simulink model "MVP2_BVA_Control_Final_Arduino1"  (R2020a)
settings: Solver=FixedStepAuto  StartTime=0.0  StopTime=inf  FixedStep=0.01  RelTol=1e-3  EnableMultiTasking=on
PreLoadFcn:
  | Time=[
  | 0
  | 0.15
  | 0.3
  | 0.45
  | 0.6
  | 0.75
  | 0.9
  | 1.05
  | 1.2
  | 1.35
  | 1.5
  | 1.65
  | 1.8
  | 1.95
  | 2.1
  | 2.25
  | 2.4
  | 2.55
  | 2.7
  | 2.85
  | 3]
  | Output=[
  | 1
  | 1
  | 1
  | 1
  | 1
  | 1
  | 1
  | 1
  | 1
  | 1
  | 1
  | 0
  | 0
  | 0
  | 0
  | 0
  | 0
  | 0
  | 0
  | 0
  | 0];
InitFcn:
  | k=3/6;
libraries: arduinolib x13
settings Model: SILPILModeSetting=veronly  ExtModeTrigDuration=2  Creator=drlee  LastModifiedBy=drlee
settings SolverCC: AutoInsertRateTranBlk=on
settings OptimizationCC: EnhancedBackFolding=on  PassReuseOutputArgsAs=Individual arguments  ZeroExternalMemoryAtStartup=off  ZeroInternalMemoryAtStartup=off  MaxStackSize=64  OptimizeBlockOrder=speed  DifferentSizesBufferReuse=on  OptimizationCustomize=off  EfficientTunableParamExpr=on
settings DebuggingCC: ParameterPrecisionLossMsg=none  ParameterTunabilityLossMsg=error
settings HardwareCC: ProdBitPerInt=16  ProdBitPerPointer=16  ProdBitPerSizeT=16  ProdBitPerPtrDiffT=16  ProdLargestAtomicFloat=None  ProdWordSize=8  ProdHWDeviceType=Atmel->AVR  UseEmbeddedCoderFeatures=off  UseSimulinkCoderFeatures=off
settings SFSimCC: MATLABDynamicMemAlloc=off
settings RTWCC: SystemTargetFile=ert.tlc  HardwareBoard=Arduino Uno  TLCOptions=-aInlineSetEventsForThisBaseRateFcn=TLC_FALSE -aSuppressMultiTaskScheduler=TLC_FALSE -aRateBasedStepFcn=1  TemplateMakefile=ert_default_tmf  RTWVerbose=off  Toolchain=Arduino AVR  BuildConfiguration=Faster Runs
settings CodeAppCC: ForceParamTrailComments=on  OperatorAnnotations=on  SimulinkDataObjDesc=on  SFDataObjDesc=on  InsertBlockDesc=on
settings ERTTargetCC: SupportContinuousTime=on  SupportNonInlinedSFcns=on  SupportVariableSizeSignals=on  ExtModeStaticAllocSize=250  ExtModeMexArgs='127.0.0.1' 0 17725  ERTSrcFileBannerTemplate=codertarget_code_template.cgt  ERTHdrFileBannerTemplate=codertarget_code_template.cgt  ERTDataSrcFileTemplate=codertarget_code_template.cgt  ERTDataHdrFileTemplate=codertarget_code_template.cgt

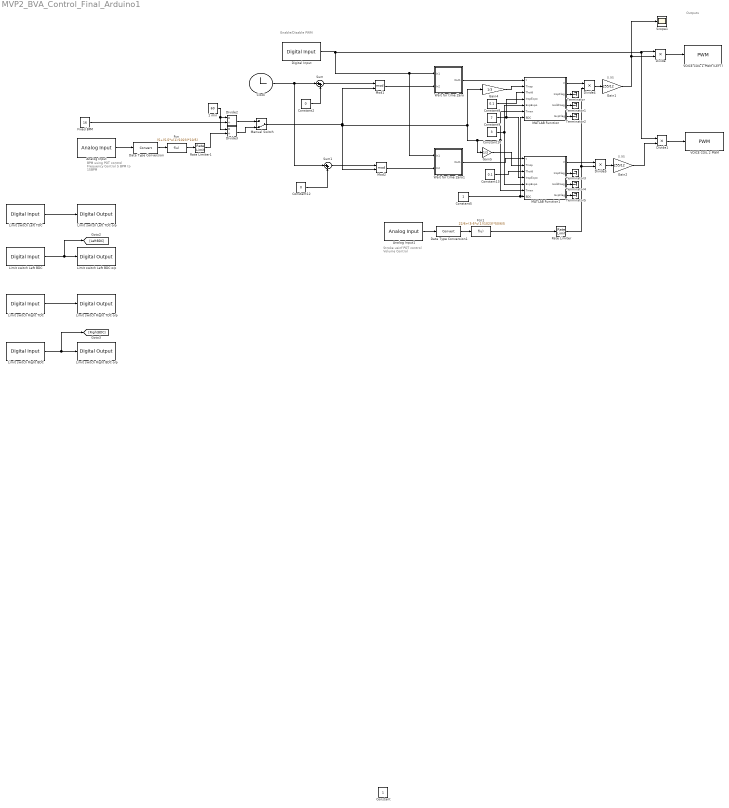
== system MVP2_BVA_Control_Final_Arduino1 ==
  note: 0.95
  note: BPM using POT control
      | Frequency Control
      | 5 BPM to 15BPM
  note: Outputs
  note: Enable/Disable PWM
  note: Stroke usinf POT control
      | Volume Control
  note: 0.95
  1 min : Constant  Value=60
  Analog Input : arduinolib/Analog Input  pinNumber=4  ReadResultsOnly=off  ConversionTriggerSource=Software  ExternalTriggerType=uint32( 0 )  OutputDataType=uint16  EnableConversionCompleteNotify=off  EnableOuputStatus=off  SampleTime=-1  blockPlatform=arduino
  Analog Input1 : arduinolib/Analog Input  pinNumber=5  ReadResultsOnly=off  ConversionTriggerSource=Software  ExternalTriggerType=uint32( 0 )  OutputDataType=uint16  EnableConversionCompleteNotify=off  EnableOuputStatus=off  SampleTime=-1  blockPlatform=arduino
  Clock : Clock
  Constant10 : Constant  Value=3
  Constant12 : Constant  Value=0
  Constant13 : Constant  Value=0.1
  Constant2 : Constant  Value=0
  Constant5 : Constant
  Constant8 : Constant  Value=0.1
  Constant9 : Constant  Value=7
  Data Type Conversion : DataTypeConversion
  Data Type Conversion1 : DataTypeConversion
  Digital Input : arduinolib/Digital Input  pinNumber=4  Direction=input  SampleTime=-1  blockPlatform=arduino
  Divide{,1,4..5} (4 alike) : Product  Inputs=**
  Divide2 : Product  Inputs=*/
  Divide3 : Product  Inputs=*/
  Fcn : Fcn  Expr=(5+(5-5*u(1)/1023)*10/5)
  Fcn1 : Fcn  Expr=22/6+(5-5*u(1)/1023)*50/6/5
  Fixed BPM : Constant  Value=16
  Gain1 : Gain  Gain=255/12
  Gain2 : Gain  Gain=255/12
  Gain4 : Gain  Gain=1/3
  Gain5 : Gain  Gain=1/3
  Limit switch Left BDC : arduinolib/Digital Input  pinNumber=3  Direction=input  SampleTime=-1  blockPlatform=arduino
  Limit switch Left BDC o/p : arduinolib/Digital Output  pinNumber=11  Direction=output  blockPlatform=arduino
  Limit switch Left TDC : arduinolib/Digital Input  pinNumber=2  Direction=input  SampleTime=-1  blockPlatform=arduino
  Limit switch Left TDC o/p : arduinolib/Digital Output  pinNumber=10  Direction=output  blockPlatform=arduino
  Limit switch Right BDC : arduinolib/Digital Input  pinNumber=7  Direction=input  SampleTime=-1  blockPlatform=arduino
  Limit switch Right BDC o/p : arduinolib/Digital Output  pinNumber=13  Direction=output  blockPlatform=arduino
  Limit switch Right TDC : arduinolib/Digital Input  pinNumber=5  Direction=input  SampleTime=-1  blockPlatform=arduino
  Limit switch Right TDC o/p : arduinolib/Digital Output  pinNumber=12  Direction=output  blockPlatform=arduino
  MATLAB Function : MATLAB Function  TreatAsAtomicUnit=on
  MATLAB Function1 : MATLAB Function  TreatAsAtomicUnit=on
  Manual Switch : ManualSwitch  CurrentSetting=0
  Mod1 : Math  Operator=mod  SaturateOnIntegerOverflow=on
  Mod2 : Math  Operator=mod  SaturateOnIntegerOverflow=on
  Rate Limiter : RateLimiter  RisingSlewLimit=0.5  FallingSlewLimit=-0.5  SampleTimeMode=inherited
  Rate Limiter1 : RateLimiter  RisingSlewLimit=0.2  FallingSlewLimit=-0.2  SampleTimeMode=inherited
  Scope1 : Scope
  Sum : Sum  Inputs=|++
  Sum1 : Sum  Inputs=|++
  Terminator{,1..5} (6 alike) : Terminator
  VOICE COIL 1 PWM (LEFT) : arduinolib/PWM  pinNumber=6  frequencyType=Default  desiredFrequency=490.2  achievableFrequency=490.2
  VOICE COIL 2 PWM : arduinolib/PWM  pinNumber=9  frequencyType=Default  desiredFrequency=490.2  achievableFrequency=490.2
  Wait for time Zero : Subsystem
  Wait for time Zero1 : Subsystem
  Constant : Constant  IOType=siggen
  wires:
  Divide4/1 -> Gain1/1
  Constant2/1 -> Sum/2
  Clock/1 -> Sum1/1, Sum/1
  Sum/1 -> Mod1/1
  Wait for time Zero/1(Out1) -> MATLAB Function/1(t)
  Mod1/1 -> Wait for time Zero/2(In2)
  Mod2/1 -> Wait for time Zero1/2(In2)
  Analog Input/1 -> Data Type Conversion/1
  Divide/1 -> VOICE COIL 1 PWM (LEFT)/1
  Divide1/1 -> VOICE COIL 2 PWM/1
  Gain4/1 -> MATLAB Function/2(Tinsp)
  Constant8/1 -> MATLAB Function/3(Thold)
  Constant9/1 -> MATLAB Function1/4(InspExpo), MATLAB Function/4(InspExpo)
  Constant10/1 -> MATLAB Function1/5(ExpExpo), MATLAB Function/5(ExpExpo)
  Gain2/1 -> Divide1/2
  Manual Switch/1 -> Mod1/2, Mod2/2, Gain5/1, MATLAB Function1/6(Tmax), MATLAB Function/6(Tmax), Gain4/1
  Wait for time Zero1/1(Out1) -> MATLAB Function1/1(t)
  Sum1/1 -> Mod2/1
  Constant12/1 -> Sum1/2
  Constant13/1 -> MATLAB Function1/3(Thold)
  MATLAB Function/1(V) -> Divide4/1
  MATLAB Function1/1(V) -> Divide5/1
  Digital Input/1 -> Divide1/1, Divide/1, Wait for time Zero1/1(In1), Wait for time Zero/1(In1)
  Gain5/1 -> MATLAB Function1/2(Tinsp)
  Analog Input1/1 -> Data Type Conversion1/1
  Limit switch Left TDC/1 -> Limit switch Left TDC o/p/1
  Limit switch Left BDC/1 -> [LeftBDC], Limit switch Left BDC o/p/1
  Limit switch Right TDC/1 -> Limit switch Right TDC o/p/1
  Limit switch Right BDC/1 -> [RightBDC], Limit switch Right BDC o/p/1
  Divide3/1 -> Manual Switch/2
  Divide2/1 -> Manual Switch/1
  1 min/1 -> Divide3/1, Divide2/1
  Fixed BPM/1 -> Divide2/2
  Fcn/1 -> Rate Limiter1/1
  Data Type Conversion/1 -> Fcn/1
  Data Type Conversion1/1 -> Fcn1/1
  Gain1/1 -> Scope1/1, Divide/2
  Divide5/1 -> Gain2/1
  Rate Limiter/1 -> Divide4/2, Divide5/2
  Rate Limiter1/1 -> Divide3/2
  Fcn1/1 -> Rate Limiter/1
  Constant5/1 -> MATLAB Function1/7(BDC), MATLAB Function/7(BDC)
  MATLAB Function/2(InspFlag) -> Terminator/1
  MATLAB Function/3(HoldFLag) -> Terminator1/1
  MATLAB Function/4(ExpFlag) -> Terminator2/1
  MATLAB Function1/2(InspFlag) -> Terminator3/1
  MATLAB Function1/3(HoldFLag) -> Terminator4/1
  MATLAB Function1/4(ExpFlag) -> Terminator5/1

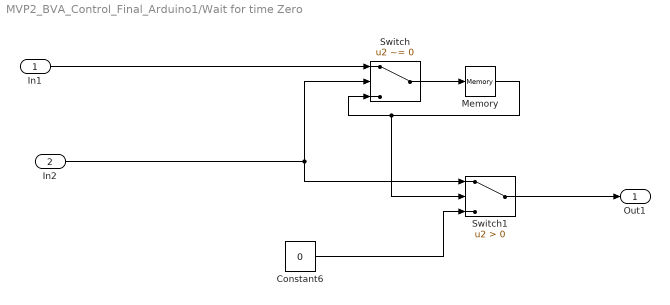
== system MVP2_BVA_Control_Final_Arduino1/Wait for time Zero ==
  In1 : Inport
  In2 : Inport  Port=2
  Constant6 : Constant  Value=0
  Memory : Memory
  Switch : Switch  Criteria=u2 ~= 0
  Switch1 : Switch  Criteria=u2 > Threshold
  Out1 : Outport
  wires:
  In2/1 -> Switch/2, Switch1/1
  Memory/1 -> Switch1/2, Switch/3
  Constant6/1 -> Switch1/3
  Switch/1 -> Memory/1
  Switch1/1 -> Out1/1
  In1/1 -> Switch/1

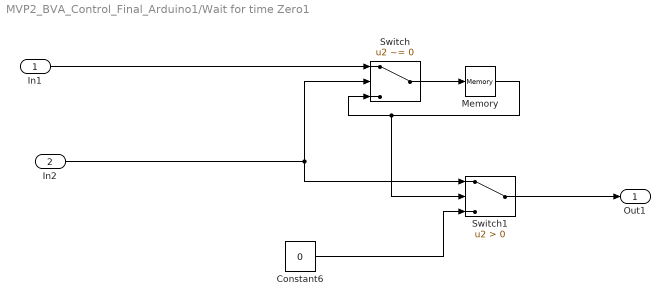
== system MVP2_BVA_Control_Final_Arduino1/Wait for time Zero1 ==
  In1 : Inport
  In2 : Inport  Port=2
  Constant6 : Constant  Value=0
  Memory : Memory
  Switch : Switch  Criteria=u2 ~= 0
  Switch1 : Switch  Criteria=u2 > Threshold
  Out1 : Outport
  wires:
  In1/1 -> Switch/1
  Switch1/1 -> Out1/1
  Switch/1 -> Memory/1
  Constant6/1 -> Switch1/3
  Memory/1 -> Switch/3, Switch1/2
  In2/1 -> Switch1/1, Switch/2

== matlab function MVP2_BVA_Control_Final_Arduino1/MATLAB Function1 ==
  data: t input; V output; Tinsp input; Thold input; InspExpo input; ExpExpo input; Tmax input; InspFlag output; HoldFLag output; ExpFlag output; BDC input
function [V,InspFlag, HoldFLag, ExpFlag] = fcn(t,Tinsp,Thold,InspExpo,ExpExpo,Tmax,BDC)
Texp=Tmax-Tinsp;
T1=Tinsp;
T2=Tinsp+Thold;
T3=Tmax;

if t< T1
    if BDC>0
        V = (1-exp(-t/Tinsp*InspExpo));
    else
        V=0;
    end
    InspFlag=1;
    HoldFLag=0;
    ExpFlag=0;
elseif t>=T2 && t< T3
    V=exp(-(t-Tinsp-Thold)/(Texp-Thold)*ExpExpo);
    InspFlag=0;
    HoldFLag=1;
    ExpFlag=0;
%     V=-1/(T3-T2)*(t-T3);
% elseif t>Tinsp && t<Thold
%     V=1;
else
    V=1;
    InspFlag=0;
    HoldFLag=0;
    ExpFlag=1;
end

== matlab function MVP2_BVA_Control_Final_Arduino1/MATLAB Function ==
  data: t input; V output; Tinsp input; Thold input; InspExpo input; ExpExpo input; Tmax input; InspFlag output; HoldFLag output; ExpFlag output; BDC input
function [V,InspFlag, HoldFLag, ExpFlag] = fcn(t,Tinsp,Thold,InspExpo,ExpExpo,Tmax,BDC)
Texp=Tmax-Tinsp;
T1=Tinsp;
T2=Tinsp+Thold;
T3=Tmax;

if t< T1
    if BDC>0
        V = (1-exp(-t/Tinsp*InspExpo));
    else
        V=0;
    end
    InspFlag=1;
    HoldFLag=0;
    ExpFlag=0;
elseif t>=T2 && t< T3
    V=exp(-(t-Tinsp-Thold)/(Texp-Thold)*ExpExpo);
    InspFlag=0;
    HoldFLag=1;
    ExpFlag=0;
%     V=-1/(T3-T2)*(t-T3);
% elseif t>Tinsp && t<Thold
%     V=1;
else
    V=1;
    InspFlag=0;
    HoldFLag=0;
    ExpFlag=1;
end
